simulink model "planar_dynamics_block"  (R2020a)
settings: Solver=VariableStepAuto  StartTime=0.0  StopTime=10.0  RelTol=1e-3
settings Model: Creator=ursk  LastModifiedBy=Karthik

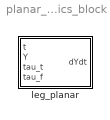
== system planar_dynamics_block ==
  leg_planar : MATLAB Function  TreatAsAtomicUnit=on

== matlab function planar_dynamics_block/leg_planar ==
  data: t input; dYdt output; Y input; tau_t input; tau_f input
function dYdt = leg_planar(t,Y,tau_t,tau_f)
%#codegen

%    This function was generated by the Symbolic Math Toolbox version 8.5.
%    16-Aug-2021 12:56:33

t2 = Y(1);
t3 = Y(2);
t4 = Y(3);
t5 = Y(4);
t6 = Y(6);
t14 = sqrt(2.0);
t22 = sqrt(7.45e+2);
t23 = sqrt(8.09e+2);
t24 = 3.860051813123757e+1;
t25 = 4.022437072223753e+1;
t27 = 7.763407756906757e+2;
t28 = 1.097911654005002e+3;
t33 = tau_f.*5.985e+11;
t34 = tau_t.*5.985e+11;
t38 = 7.994124630883609e+5;
t57 = cos(1.470783553884025e-1);
t58 = sin(1.470783553884025e-1);
t7 = cos(t2);
t8 = cos(t4);
t9 = sin(t2);
t10 = sin(t4);
t11 = t4.*2.0;
t12 = t3.^2;
t13 = t5.^2;
t15 = -t2;
t16 = -t4;
t19 = t2+t4;
t31 = t5.*2.6334e+9;
t32 = t6.*2.6334e+9;
t36 = t24.*5.0274e+5;
t39 = t23.*4.507303881061812e-4;
t47 = t23.*9.016089599069681e-4;
t59 = t2+1.470783553884025e-1;
t60 = t4+1.470783553884025e-1;
t61 = t4+2.94156710776805e-1;
t68 = t4-1.470783553884025e-1;
t89 = t22.*t57.*4.9514004e+7;
t90 = t27.*t58.*2.1384e+4;
t17 = cos(t11);
t18 = sin(t11);
t20 = cos(t19);
t21 = sin(t19);
t26 = t2+t16;
t35 = -t31;
t40 = atan(t39);
t41 = t7.*t14.*6.16484925e+9;
t42 = t9.*t14.*6.16484925e+9;
t49 = atan(t47);
t50 = t7.*t22.*2.9185726095e+10;
t51 = t8.*t23.*tau_t.*1.62e+10;
t52 = t5.*t8.*t23.*7.128e+7;
t54 = t10.*t12.*t23.*6.0598125e+8;
t55 = t10.*t13.*t23.*1.2119625e+9;
t56 = t3.*t5.*t10.*t23.*1.81794375e+9;
t62 = cos(t59);
t63 = cos(t60);
t64 = cos(t61);
t65 = sin(t59);
t66 = sin(t60);
t67 = sin(t61);
t69 = t11+1.470783553884025e-1;
t70 = t11+2.94156710776805e-1;
t71 = sin(t68);
t72 = t19+1.470783553884025e-1;
t73 = t19+2.94156710776805e-1;
t80 = t11+t59;
t86 = t15+t60;
t91 = -t89;
t92 = -t90;
t29 = cos(t26);
t30 = sin(t26);
t37 = t17.*5.307849e+8;
t43 = -t41;
t44 = -t42;
t45 = t12.*t18.*6.63481125e+9;
t48 = t3.*t5.*t18.*6.63481125e+9;
t53 = -t51;
t74 = cos(t69);
t75 = cos(t70);
t76 = sin(t69);
t77 = sin(t70);
t78 = cos(t72);
t79 = sin(t72);
t81 = t2+t70;
t82 = cos(t80);
t84 = sin(t80);
t87 = cos(t86);
t88 = sin(t86);
t93 = t62.*6.0716547405e+11;
t94 = t23.*t65.*2.622213e+8;
t96 = t22.*t66.*tau_t.*2.64e+8;
t97 = t5.*t22.*t66.*1.1616e+6;
t100 = t40+t69;
t102 = t5.*t27.*t63.*3.1856e+6;
t105 = t12.*t22.*t63.*9.87525e+6;
t106 = t13.*t22.*t63.*1.97505e+7;
t109 = t3.*t5.*t22.*t63.*2.962575e+7;
t110 = t27.*t63.*tau_t.*7.24e+8;
t115 = t12.*t27.*t66.*2.7082125e+7;
t116 = t13.*t27.*t66.*5.416425e+7;
t117 = t49+t70;
t126 = t3.*t5.*t27.*t66.*8.1246375e+7;
t46 = -t45;
t83 = cos(t81);
t85 = sin(t81);
t95 = t82.*5.8176973845e+11;
t99 = -t97;
t101 = t12.*t77.*9.8709866425e+9;
t104 = cos(t100);
t107 = t3.*t5.*t77.*9.8709866425e+9;
t108 = t23.*t84.*2.622213e+8;
t111 = t12.*t23.*t75.*8.89977e+6;
t112 = -t110;
t118 = t12.*t27.*t74.*2.673e+5;
t120 = t3.*t5.*t23.*t75.*8.89977e+6;
t123 = t12.*t22.*t76.*5.9303745e+8;
t124 = cos(t117);
t125 = t3.*t5.*t27.*t74.*2.673e+5;
t128 = t3.*t5.*t22.*t76.*5.9303745e+8;
t98 = -t95;
t103 = -t101;
t113 = t22.*t83.*2.5995806433e+10;
t114 = t27.*t85.*2.3438052e+7;
t119 = -t111;
t122 = -t118;
t127 = -t123;
t129 = t124.*7.89938549e+8;
t130 = t38.*t104.*1.62e+3;
t121 = -t113;
t131 = t36+t37+t91+t92+t129+t130-1.606683691e+9;
t132 = 1.0./t131;
dYdt = [t3;(t132.*(t32-t33+t34+t35+t43+t44+t46+t48+t50+t52+t53+t54+t55+t56+t93+t94+t96+t98+t99+t102+t103+t105+t106+t107+t108+t109+t112+t114+t115+t116+t119+t120+t121+t122+t125+t126+t127+t128))./2.5e+1;t5;(t132.*(t5.*6.9376912e+9-t32+t33+t41+t42-t50-t55+t79.*2.2600497744e+10-t88.*9.06832476e+9-t93-t94+t95-t106-t108+t113-t114-t116-tau_t.*1.576748e+12-t8.*t12.*1.991385e+8-t5.*t24.*7.392e+5+t12.*t18.*1.32696225e+10+t13.*t18.*1.32696225e+10+t21.*t22.*5.244426e+8-t20.*t25.*8.343405e+7-t21.*t25.*8.343405e+7-t20.*t27.*6.913107e+8+t22.*t30.*2.622213e+8-t25.*t29.*8.343405e+7-t25.*t30.*8.343405e+7+t27.*t29.*1.46605545e+9-t12.*t64.*1.991385e+8+t12.*t77.*1.9741973285e+10+t13.*t77.*1.9741973285e+10-t23.*t78.*4.5889300404e+10-t24.*t78.*1.359666e+6-t24.*t79.*4.078998e+6+t28.*t78.*1.1186343e+7-t28.*t79.*3.728781e+6+t23.*t87.*2.486919366e+10+t24.*t87.*1.359666e+6+t24.*t88.*1.359666e+6-t28.*t87.*3.728781e+6+t28.*t88.*3.728781e+6+t24.*tau_t.*1.68e+8-t27.*cos(t73).*7.1912205e+8+t23.*cos(t26+1.470783553884025e-1).*1.60908525e+10+t22.*sin(t73).*2.622213e+8+t3.*t5.*t8.*1.991385e+8+t3.*t5.*t18.*1.32696225e+10-t5.*t8.*t23.*1.4256e+8+t6.*t8.*t23.*7.128e+7-t10.*t12.*t23.*2.1425796e+9+t10.*t12.*t28.*1.701e+5+t3.*t5.*t64.*1.991385e+8+t5.*t22.*t57.*1.4256e+8+t3.*t5.*t77.*1.9741973285e+10+t12.*t14.*t63.*2.06514e+6+t5.*t22.*t66.*2.3232e+6-t6.*t22.*t66.*1.1616e+6-t5.*t27.*t63.*6.3712e+6+t6.*t27.*t63.*3.1856e+6-t12.*t22.*t63.*2.6016342e+7-t12.*t23.*t67.*5.4612225e+8+t12.*t25.*t66.*5.66349e+6-t12.*t27.*t66.*8.7750347e+7+t12.*t22.*t76.*1.1860749e+9+t12.*t23.*t75.*1.779954e+7-t12.*t27.*t71.*1.64025e+7+t13.*t22.*t76.*1.1860749e+9+t13.*t23.*t75.*1.779954e+7+t12.*t27.*t74.*5.346e+5+t13.*t27.*t74.*5.346e+5-t8.*t23.*tau_f.*1.62e+10+t8.*t23.*tau_t.*3.24e+10+t22.*t66.*tau_f.*2.64e+8-t27.*t63.*tau_f.*7.24e+8-t22.*t57.*tau_t.*3.24e+10-t22.*t66.*tau_t.*5.28e+8+t27.*t63.*tau_t.*1.448e+9-t3.*t5.*t10.*t23.*2.813454e+8-t3.*t5.*t10.*t28.*1.701e+5-t3.*t5.*t14.*t63.*2.06514e+6-t3.*t5.*t22.*t63.*1.3484658e+7+t3.*t5.*t23.*t67.*5.4612225e+8-t3.*t5.*t25.*t66.*5.66349e+6-t3.*t5.*t27.*t66.*2.0578153e+7+t3.*t5.*t22.*t76.*1.1860749e+9+t3.*t5.*t23.*t75.*1.779954e+7+t3.*t5.*t27.*t71.*1.64025e+7+t3.*t5.*t27.*t74.*5.346e+5))./2.5e+1;t6;(t132.*(t6.*9.1001003005e+10+t34+t35+t43+t44+t46+t48+t50+t52+t53+t54+t55+t56+t93+t94+t96+t98+t99+t102+t103+t105+t106+t107+t108+t109+t112+t114+t115+t116+t119+t120+t121+t122+t125+t126+t127+t128-tau_f.*2.06820461375e+13-t6.*t17.*2.91931695e+10-t6.*t24.*2.76507e+7-t6.*t75.*4.3432341227e+10+t17.*tau_f.*6.63481125e+12+t24.*tau_f.*6.28425e+9+t75.*tau_f.*9.8709866425e+12+t6.*t22.*t57.*2.72327022e+9+t6.*t27.*t58.*1.17612e+6-t6.*t22.*t74.*2.60936478e+9+t6.*t23.*t77.*3.9158988e+7+t6.*t27.*t76.*1.17612e+6-t22.*t57.*tau_f.*6.1892505e+11-t27.*t58.*tau_f.*2.673e+8+t22.*t74.*tau_f.*5.9303745e+11-t23.*t77.*tau_f.*8.89977e+9-t27.*t76.*tau_f.*2.673e+8))./2.5e+1];
